simulink model "soc_WLAN_fpga"  (R2024b)
settings: Solver=FixedStepDiscrete  StartTime=0.0  StopTime=stopTime  RelTol=1e-3
PreLoadFcn:
  | addpath(fullfile(matlabroot,'toolbox','whdl','whdlexamples','whdlexamples'));
InitFcn:
  | addpath(fullfile(matlabroot,'toolbox','whdl','whdlexamples','whdlexamples'));
model workspace (MAT data in the model file):
  socvcb : containers.Map (value not decoded)
undefined symbols (not defined in the file): Add, bitRatePerOfdmSym, chanBW, coe, cpLen, dataUpsampleFactor, DelayValMaxNsdMinusLastPilotSc, DescramblerInitialSeed, designMultirateFIR, fftLen, filterLatency, filterUpsampleFactor, Fs, Hd, HT_MFMCS0, HT_MFMCS1, HT_MFMCS2, HT_MFMCS3, HT_MFMCS4, HT_MFMCS5, HT_MFMCS6, HT_MFMCS7, HTUnUsedScInd, inputSamplingRate, interp_coeff, maxPilotRefCounterVale, maxPilotsRef, maxPilotsRefNonHT, Ncol_HT, Ncol_NonHT, noDataSubCarriers, Non_HTMCS0, Non_HTMCS1, Non_HTMCS2, Non_HTMCS3, Non_HTMCS4, Non_HTMCS5, Non_HTMCS6, Non_HTMCS7, Nrow_HT, Nrow_NonHT, numDSC_HT, numDSC_HT_vhtSigB, numDSC_NonHT, numDscHT, numDscNonHT, numOfBitsPerOFDMSym, numOfDataBitsPerOFDMSym, numPilots, numScHT, numSCS_HT, numSCS_NonHT, pnSeq, QAM, rxDownsampleFactor, secondPIdx_HT, secondPIdx_NonHT, Shift, VHTMCS0, VHTMCS1 ... (+7)
libraries: hdlsllib x267, simulink x210, dspsigops x22, whdlutilities x10, whdlmod x9, dsphdlfiltering2 x5, dsphdlmathfun2 x4, whdledac x3, hwlogicconnlib x2, commhdlcrc x2, dsphdlsigops2 x2
(part 14 of 14)

== matlab function soc_WLAN_fpga/WLAN/WLAN HDL/WLAN_Tx_Rx/WLAN_Rx/WLANHDLReceiver/FrameFormatDetectionAndSignalRecovery/CRCCheckAndBitInterpretation/LSigBitRecover ==
  data: bit input; failCheck output; validIn input; MCS output; PSDULen output; rst input
function [failCheck,MCS,PSDULen] = LSigBitRecover(bit,validIn,rst)
%#codegen
persistent bitXORVal;
persistent countVal;
persistent mcsBitReg;
persistent psduLenReg;
persistent Pow2Reg;
persistent Pow2Reg1;
persistent psduLenRegDelay;
persistent MCSDelay;

if isempty(bitXORVal)||rst
    bitXORVal = false;
    countVal = uint8(0);
    mcsBitReg = uint16(0); % default for MCS 0
    psduLenReg = fi(0,0,17,0);
    psduLenRegDelay = fi(0,0,17,0);
    Pow2Reg = uint16([1,2,4,8,16,32,64,128,256,512,1024,2048]); % Starts with LSB
    Pow2Reg1 = uint16([4,2,1]);
    MCSDelay = uint8(0);
end
failCheck = false;
MCS = uint8(MCSDelay);
PSDULen = fi(psduLenRegDelay,0,17,0);

if validIn
    countVal(:) = countVal + 1;    
    if countVal <= 17
        if countVal <= 3
            if bit == 1
                mcsBitReg(:) = mcsBitReg + Pow2Reg1(countVal) ; 
            end
        end
        if countVal == 3
            switch(mcsBitReg)
                case 6 % [1 1 0]
                    MCS = uint8(0);
                case 7 % [1 1 1]
                    MCS = uint8(1);
                case 2 % [0 1 0]
                    MCS = uint8(2);
                case 3 % [0 1 1]
                    MCS = uint8(3);
                case 4 % [1 0 0]
                    MCS = uint8(4);
                case 5 % [1 0 1]
                    MCS = uint8(5);
                case 0 % [0 0 0]
                    MCS = uint8(6);
                case 1 % [0 0 1]
                    MCS = uint8(7);
                otherwise
                    MCS = uint8(0);
            end
            MCSDelay = MCS;
        end
        if countVal >= 6
            if bit == 1
            psduLenReg(:) = psduLenReg +  Pow2Reg(countVal-5);
            end
        end
        if countVal == 4
            if bit == 0
            failCheck = true;
            end
        end
        bitXORVal = bitxor(bitXORVal,bit);
        if countVal == 17
            PSDULen = fi(psduLenReg,0,17,0);
            psduLenRegDelay(:) = psduLenReg;
        else
            PSDULen = fi(psduLenRegDelay,0,17,0);
        end
    elseif countVal == 18
        if bitXORVal ~= bit
            failCheck = true;
        end
        PSDULen = fi(psduLenRegDelay,0,17,0);
    end
end


end

== matlab function soc_WLAN_fpga/WLAN/WLAN HDL/WLAN_Tx_Rx/WLAN_Rx/WLANHDLReceiver/FrameFormatDetectionAndSignalRecovery/FormatIdentification/frameFormatMapping ==
  data: symbNum input; frameFormat output; MCS input; isQBPSK input; formatDetected output; reset input
function [frameFormat,formatDetected] = frameFormatMapping(symbNum,MCS,isQBPSK,reset)
%#codegen

persistent NonHTFlag;
persistent HTMMFlag;
persistent VHTFlag;


if isempty(NonHTFlag) || reset
    NonHTFlag = false;
    HTMMFlag = false;
    VHTFlag = false;
    
end

if symbNum == 4 && MCS ~= 0
    NonHTFlag = true;
end

if ~NonHTFlag
    if symbNum == 5 && isQBPSK == true && MCS == 0
        HTMMFlag = true;
    end
    
    if ~HTMMFlag
        if symbNum == 6 && isQBPSK == true && MCS == 0
            VHTFlag = true;
        end
    end
end

if NonHTFlag
    frameFormat = fi(0,0,2,0);
elseif HTMMFlag
    frameFormat = fi(1,0,2,0);
elseif VHTFlag
    frameFormat = fi(2,0,2,0);
else
    frameFormat = fi(0,0,2,0);
end
if symbNum == 6
    formatDetected = (NonHTFlag || HTMMFlag || VHTFlag) ;
else
    formatDetected = false;
end
if reset
    frameFormat = fi(0,0,2,0);
    formatDetected = false;
end

== matlab function soc_WLAN_fpga/WLAN/WLAN HDL/WLAN_Tx_Rx/WLAN_Rx/WLANHDLReceiver/FrameFormatDetectionAndSignalRecovery/SignalBitRecovery/Deinterleaver Block/Generate Ready/MATLAB Function1 ==
  data: trigger input; out output; nClocks parameter
function out = holdPulse(trigger,nClocks)
%#codegen

 persistent count state;
 if isempty(count)
     count = fi(0,0,nextpow2(nClocks+2),0,hdlfimath);
     state = false;
 end
 
 
 %% Executes in current clock cycle
 if trigger
     state = true;
     count(:) = 0;
 end
 
 if(state && ~trigger)
     count(:) = count +1;
 end
 
 if(count(:) == (nClocks))
    state = false;
 end
     
 out = state;
 
end

== matlab function soc_WLAN_fpga/WLAN/WLAN HDL/WLAN_Tx_Rx/WLAN_Rx/WLANHDLReceiver/FrameFormatDetectionAndSignalRecovery/SignalBitRecovery/Deinterleaver Block/Read Logic/MATLAB Function ==
  data: trigger input; out output; nClocks parameter
function out = holdPulse(trigger,nClocks)
%#codegen

 persistent count state;
 if isempty(count)
     count = fi(0,0,nextpow2(nClocks+1),0,hdlfimath);
     state = false;
 end
 
 %% Executes in next clock cycle
 if(count(:) == (nClocks))
    state = false;
 end
     
 out = state;
 
 
 %% Executes in current clock cycle
 if trigger
     state = true;
     count(:) = 0;
 end
 
 if(state && ~trigger)
     count(:) = count +1;
 end
 
end

== matlab function soc_WLAN_fpga/WLAN/WLAN HDL/WLAN_Tx_Rx/WLAN_Rx/WLANHDLReceiver/FrameFormatDetectionAndSignalRecovery/SignalBitRecovery/sampleParallel ==
  data: dataIn input; dataOut output; startOut output; endOut output; validIn input; validOut output; rst input
function [dataOut,startOut,endOut,validOut] = sampleParallel(dataIn,validIn,rst)
%#codegen

persistent dataBuff
persistent vecCount;
persistent sampleCount;
persistent signalBitLen;
if isempty(dataBuff)||rst
    dataBuff = cast(zeros(2,1),'like',dataIn);
    vecCount = uint8(0);
    sampleCount = uint8(0);
    signalBitLen = uint8(48); % initializing with L-Sig length
end

if validIn 
    sampleCount(:) = sampleCount + 1;
    vecCount(:) = vecCount + 1;
    dataBuff(vecCount) = dataIn;
end
if sampleCount == 2 && validIn
    startOut = true;
    endOut = false;
elseif sampleCount == signalBitLen && validIn
    startOut = false;
    endOut = true;
    sampleCount(:)=0;
    signalBitLen =  uint8(96); % Updating length for HT/VHT signal fields
else
    startOut = false;
    endOut = false;
end
if vecCount == 2
    dataOut = dataBuff;
    validOut = true;
    vecCount(:) = 0;
else
    dataOut = cast(zeros(2,1),'like',dataIn);
    validOut = false;
end
